simulink model "linear_simulation"  (R2023a)
settings: Solver=VariableStepAuto  StartTime=0.0  StopTime=20  MaxStep=5e-5  RelTol=1e-3
values from neighbouring files (symbols this model uses):
  a1 = Ax0(1, 1)    [linearmodel.m]
  a2 = Ax0(1, 2)    [linearmodel.m]
  a3 = Ax0(1, 3)    [linearmodel.m]
  a4 = bx0(1)    [linearmodel.m]
  b1 = Ax0(3, 1)    [linearmodel.m]
  b2 = Ax0(3, 2)    [linearmodel.m]
  b3 = Ax0(3, 3)    [linearmodel.m]
  b4 = bx0(3)    [linearmodel.m]
libraries: cstblocks x5
settings Model: Creator=gabri  LastModifiedBy=gabri

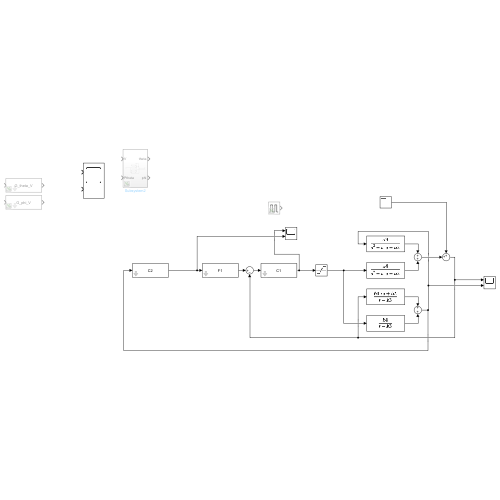
[thumbnail: Simulink's stored preview of the top-level diagram]
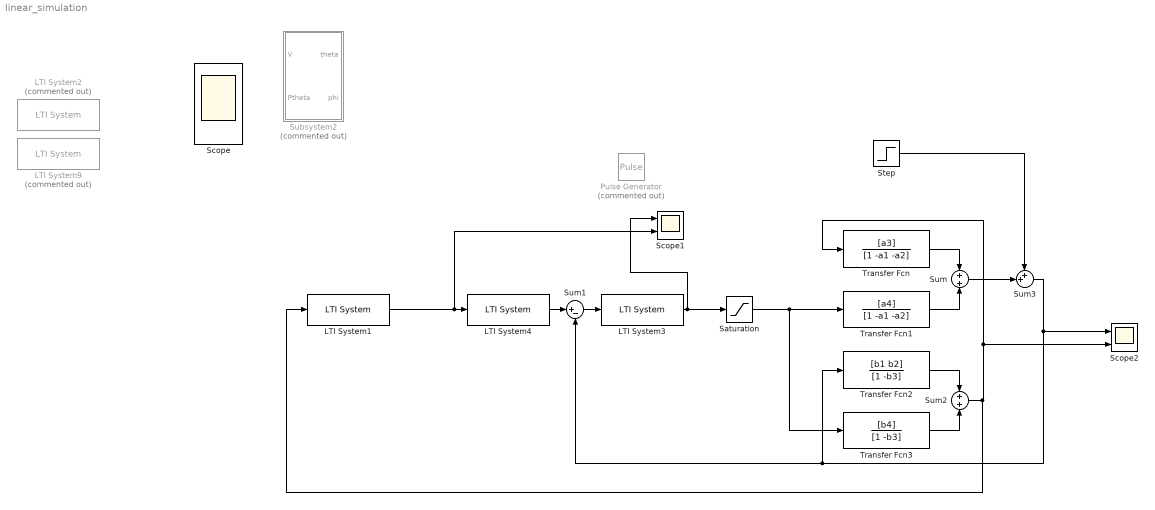
== system linear_simulation ==
  LTI System1 : cstblocks/LTI System  sys=C2  IC=[]
  LTI System2 : cstblocks/LTI System  Commented=on  sys=G_theta_V  IC=[]
  LTI System3 : cstblocks/LTI System  sys=C1  IC=[]
  LTI System4 : cstblocks/LTI System  sys=F1  IC=[]
  LTI System9 : cstblocks/LTI System  Commented=on  sys=G_phi_V  IC=[]
  Pulse Generator : DiscretePulseGenerator  Commented=on  PulseType=Time based  Amplitude=0.2  PulseWidth=10  PhaseDelay=2
  Saturation : Saturate  UpperLimit=100  LowerLimit=-100
  Scope : Scope  NumInputPorts=2
  Scope1 : Scope  NumInputPorts=2
  Scope2 : Scope  NumInputPorts=2
  Step : Step  Time=0  Before=0.1  After=0  SampleTime=0
  Subsystem2 : Subsystem  Commented=on
  Sum : Sum
  Sum1 : Sum  Inputs=|+-
  Sum2 : Sum
  Sum3 : Sum  Inputs=++|
  Transfer Fcn : TransferFcn  Numerator=[a3]  Denominator=[1 -a1 -a2]
  Transfer Fcn1 : TransferFcn  Numerator=[a4]  Denominator=[1 -a1 -a2]
  Transfer Fcn2 : TransferFcn  Numerator=[b1 b2]  Denominator=[1 -b3]
  Transfer Fcn3 : TransferFcn  Numerator=[b4]  Denominator=[1 -b3]
  wires:
  LTI System4/1 -> Sum1/1
  Sum1/1 -> LTI System3/1
  Transfer Fcn1/1 -> Sum/2
  Sum/1 -> Sum3/2
  Transfer Fcn2/1 -> Sum2/1
  Transfer Fcn/1 -> Sum/1
  Transfer Fcn3/1 -> Sum2/2
  Sum3/1 -> Sum1/2, Transfer Fcn2/1, Scope2/1
  LTI System3/1 -> Scope1/1, Saturation/1
  Sum2/1 -> LTI System1/1, Scope2/2, Transfer Fcn/1
  LTI System1/1 -> Scope1/2, LTI System4/1
  Saturation/1 -> Transfer Fcn3/1, Transfer Fcn1/1
  Step/1 -> Sum3/1

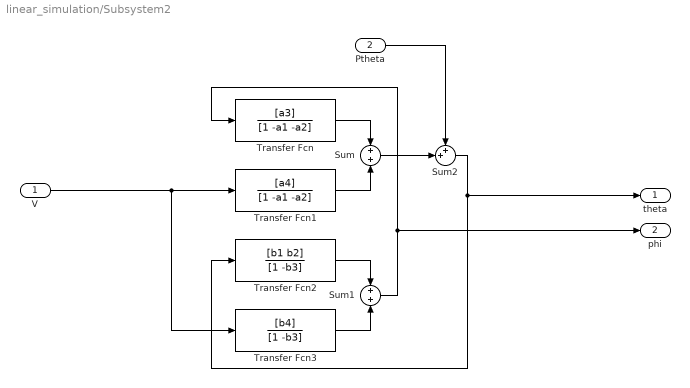
== system linear_simulation/Subsystem2 ==
  V : Inport
  Ptheta : Inport  Port=2
  Sum : Sum
  Sum1 : Sum
  Sum2 : Sum  Inputs=++|
  Transfer Fcn : TransferFcn  Numerator=[a3]  Denominator=[1 -a1 -a2]
  Transfer Fcn1 : TransferFcn  Numerator=[a4]  Denominator=[1 -a1 -a2]
  Transfer Fcn2 : TransferFcn  Numerator=[b1 b2]  Denominator=[1 -b3]
  Transfer Fcn3 : TransferFcn  Numerator=[b4]  Denominator=[1 -b3]
  theta : Outport
  phi : Outport  Port=2
  wires:
  Sum2/1 -> Transfer Fcn2/1, theta/1
  Ptheta/1 -> Sum2/1
  Sum/1 -> Sum2/2
  Transfer Fcn2/1 -> Sum1/1
  Transfer Fcn/1 -> Sum/1
  Sum1/1 -> phi/1, Transfer Fcn/1
  Transfer Fcn3/1 -> Sum1/2
  V/1 -> Transfer Fcn1/1, Transfer Fcn3/1
  Transfer Fcn1/1 -> Sum/2
